simulink model "RLC_Block_Diagram"  (R2022a)
settings: Solver=VariableStepAuto  StartTime=0.0  StopTime=10.0  RelTol=1e-3
undefined symbols (not defined in the file): C, i_L0, L, R, u_C0
settings Model: Creator=Rohan More  LastModifiedBy=Rohan More

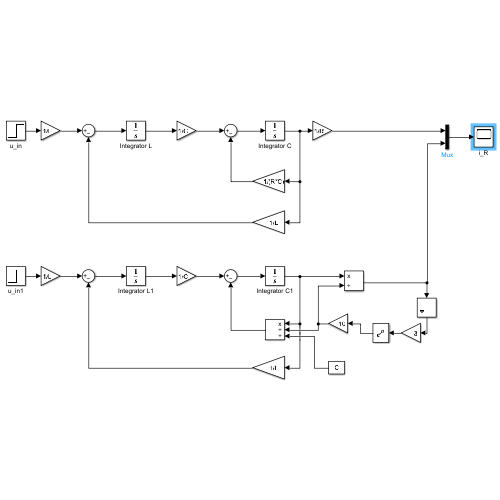
[thumbnail: Simulink's stored preview of the top-level diagram]
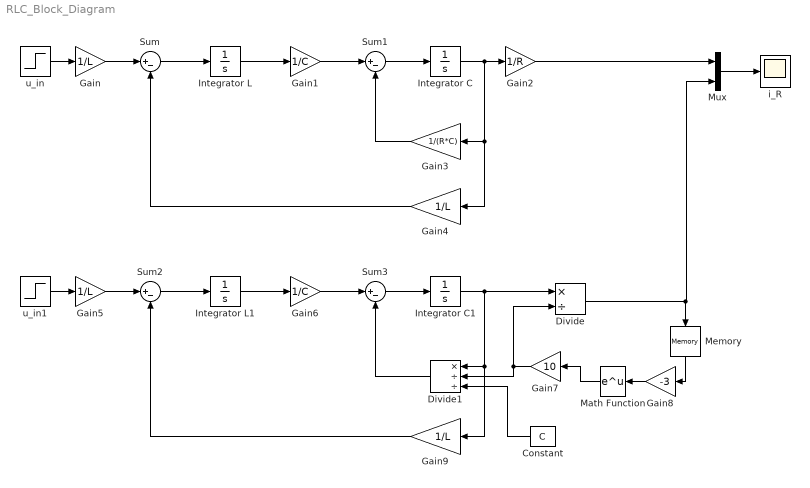
== system RLC_Block_Diagram ==
  Constant : Constant  Value=C
  Divide : Product  Inputs=*/
  Divide1 : Product  Inputs=*//
  Gain{,4..5,9} (4 alike) : Gain  Gain=1/L
  Gain1 : Gain  Gain=1/C
  Gain2 : Gain  Gain=1/R
  Gain3 : Gain  Gain=1/(R*C)
  Gain6 : Gain  Gain=1/C
  Gain7 : Gain  Gain=10
  Gain8 : Gain  Gain=-3
  Integrator C : Integrator  InitialCondition=u_C0
  Integrator C1 : Integrator  InitialCondition=u_C0
  Integrator L : Integrator  InitialCondition=i_L0
  Integrator L1 : Integrator  InitialCondition=i_L0
  Math Function : Math
  Memory : Memory
  Mux : Mux  Inputs=2
  Sum{,1..3} (4 alike) : Sum  Inputs=|+-
  i_R : Scope
  u_in : Step  SampleTime=0
  u_in1 : Step  SampleTime=0
  wires:
  Gain/1 -> Sum/1
  Sum/1 -> Integrator L/1
  Integrator L/1 -> Gain1/1
  Gain1/1 -> Sum1/1
  Sum1/1 -> Integrator C/1
  Integrator C/1 -> Gain4/1, Gain3/1, Gain2/1
  Gain4/1 -> Sum/2
  Gain3/1 -> Sum1/2
  u_in/1 -> Gain/1
  u_in1/1 -> Gain5/1
  Sum3/1 -> Integrator C1/1
  Divide1/1 -> Sum3/2
  Gain9/1 -> Sum2/2
  Sum2/1 -> Integrator L1/1
  Integrator C1/1 -> Divide/1, Gain9/1, Divide1/1
  Gain6/1 -> Sum3/1
  Integrator L1/1 -> Gain6/1
  Gain5/1 -> Sum2/1
  Divide/1 -> Mux/2, Memory/1
  Constant/1 -> Divide1/3
  Gain7/1 -> Divide1/2, Divide/2
  Math Function/1 -> Gain7/1
  Gain8/1 -> Math Function/1
  Gain2/1 -> Mux/1
  Mux/1 -> i_R/1
  Memory/1 -> Gain8/1
